simulink model "tf_function"  (R2022b)
settings: Solver=ode5  StartTime=0.0  StopTime=t_s  FixedStep=h  RelTol=1e-3
undefined symbols (not defined in the file): A, B
settings Model: Creator=Claudia  LastModifiedBy=Claudia Yasar
settings SolverCC: AlgebraicLoopSolver=TrustRegion
settings DataIOCC: ReturnWorkspaceOutputs=off
settings DebuggingCC: UnconnectedInputMsg=warning  UnconnectedOutputMsg=warning  UnconnectedLineMsg=warning  SFMachineParentedDataDiag=warning  ArithmeticOperatorsInVariantConditions=warning
settings ModelReferenceCC: EnableRefExpFcnMdlSchedulingChecks=on
settings SFSimCC: CustomCodeUndefinedFunction=UseInterfaceOnly
settings RTWCC: DLArmComputeVersion=19.05

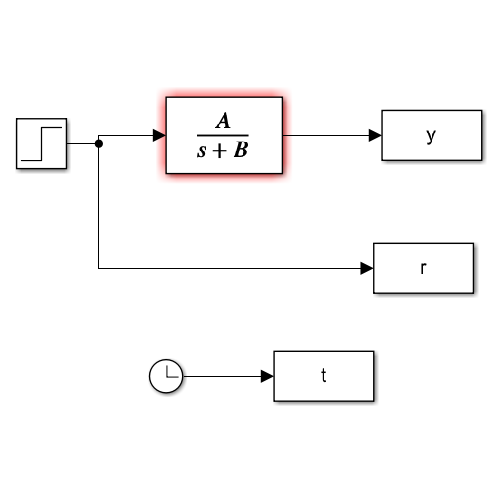
[thumbnail: Simulink's stored preview of the top-level diagram]
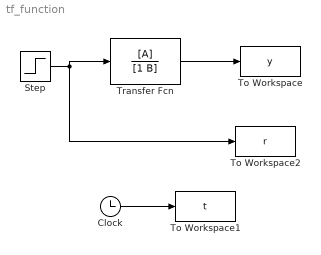
== system tf_function ==
  Clock : Clock
  Step : Step  SampleTime=0
  To Workspace : ToWorkspace  VariableName=y  SampleTime=-1
      settings: OpenFcn=figure;plot(t,y);
  To Workspace1 : ToWorkspace  VariableName=t  SampleTime=-1
  To Workspace2 : ToWorkspace  VariableName=r  SampleTime=-1
      settings: OpenFcn=figure;plot(t,y);
  Transfer Fcn : TransferFcn  Numerator=[A]  Denominator=[1 B]
  wires:
  Clock/1 -> To Workspace1/1
  Transfer Fcn/1 -> To Workspace/1
  Step/1 -> To Workspace2/1, Transfer Fcn/1
